simulink model "nonlinear_system_model"  (R2018b)
settings: Solver=ode4  StartTime=0.0  StopTime=10.0  RelTol=1e-3
values from neighbouring files (symbols this model uses):
  g = 9.81    [canonical_form.m]    (also in linear_system_open_loop_output.m; observability_and_controllability.m; realization.m; stability.m)
  i_x = 4.85e-3    (= 0.00485)    [canonical_form.m]    (also in linear_system_open_loop_output.m; observability_and_controllability.m; realization.m; stability.m)
settings Model: Creator=User  LastModifiedBy=User

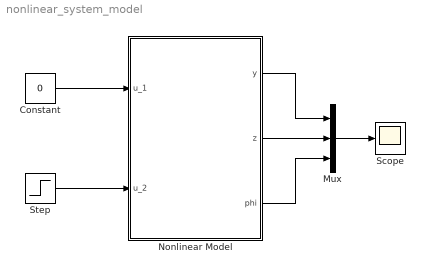
== system nonlinear_system_model ==
  Constant : Constant  Value=0
  Mux : Mux  Inputs=3
  Nonlinear Model : Subsystem
  Scope : Scope
  Step : Step  SampleTime=0
  wires:
  Mux/1 -> Scope/1
  Nonlinear Model/2(z) -> Mux/2
  Nonlinear Model/1(y) -> Mux/1
  Nonlinear Model/3(phi) -> Mux/3
  Constant/1 -> Nonlinear Model/1(u_1)
  Step/1 -> Nonlinear Model/2(u_2)

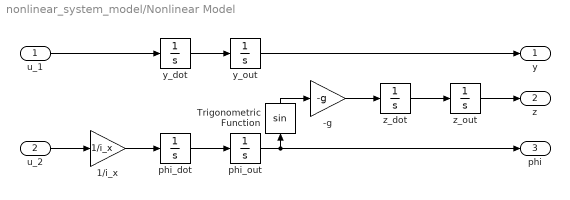
== system nonlinear_system_model/Nonlinear Model ==
  u_1 : Inport
  u_2 : Inport  Port=2
  -g : Gain  Gain=-g
  1/i_x : Gain  Gain=1/i_x
  Trigonometric Function : Trigonometry
  phi_dot : Integrator
  phi_out : Integrator
  y_dot : Integrator
  y_out : Integrator
  z_dot : Integrator
  z_out : Integrator
  y : Outport
  z : Outport  Port=2
  phi : Outport  Port=3
  wires:
  u_1/1 -> y_dot/1
  y_dot/1 -> y_out/1
  y_out/1 -> y/1
  phi_dot/1 -> phi_out/1
  1/i_x/1 -> phi_dot/1
  u_2/1 -> 1/i_x/1
  phi_out/1 -> Trigonometric Function/1, phi/1
  z_dot/1 -> z_out/1
  -g/1 -> z_dot/1
  z_out/1 -> z/1
  Trigonometric Function/1 -> -g/1
